simulink model "Day_09_Model_Predictive_Control"  (R2024a)
settings: Solver=FixedStepAuto  StartTime=0.0  StopTime=10  FixedStep=0.01  RelTol=1e-3
values from neighbouring files (symbols this model uses):
  D0 = 2700    [Day_09.m]    (also in Day_09_Method1.m; Day_09_Method2.m)
  D1 = 2700    [Day_09.m]    (also in Day_09_Method1.m; Day_09_Method2.m)
  disturbance = 0.1    [Day_09.m]    (also in Day_09_Method1.m = 0; Day_09_Method2.m = 0)
  L0 = 0.01    [Day_09.m]    (also in Day_09_Method1.m; Day_09_Method2.m)
  L1 = 0.14    [Day_09.m]    (also in Day_09_Method1.m; Day_09_Method2.m)
  limit = inf    [Day_09.m]
  M0 = L0*W0*T0*D0    (= 0.0027)    [Day_09.m]    (also in Day_09_Method1.m; Day_09_Method2.m)
  M1 = L1*W1*T1*D1    (= 0.0378)    [Day_09.m]    (also in Day_09_Method1.m; Day_09_Method2.m)
  M_c = 3    [Day_09.m]    (also in Day_09_Method1.m = 5; Day_09_Method2.m = 5)
  N_p = 10    [Day_09.m]    (also in Day_09_Method1.m = 50; Day_09_Method2.m = 50)
  Q = eye(4)    [Day_09.m]    (also in Day_09_Method1.m = [1 0; 0 1]; Day_09_Method2.m = [1 0; 0 1]; test.m = eye(20))
  R = 1    [Day_09.m]    (also in Day_09_Method1.m; Day_09_Method2.m; test.m = eye(3))
  step_size = 0.01    [Day_09.m]
  T0 = 0.01    [Day_09.m]    (also in Day_09_Method1.m; Day_09_Method2.m)
  T1 = 0.01    [Day_09.m]    (also in Day_09_Method1.m; Day_09_Method2.m)
  W0 = 0.01    [Day_09.m]    (also in Day_09_Method1.m; Day_09_Method2.m)
  W1 = 0.01    [Day_09.m]    (also in Day_09_Method1.m; Day_09_Method2.m)
  x1_d = 0    [Day_09.m]
  x2_d = 0    [Day_09.m]
  x3_d = 0    [Day_09.m]
  x4_d = 0    [Day_09.m]
undefined symbols (not defined in the file or in its folder): X, Y, Z
libraries: sm_lib x14, nesl_utility x7
settings Model: Creator=mingeun  LastModifiedBy=mingeun
settings SolverCC: ZeroCrossAlgorithm=Adaptive
settings DataIOCC: ReturnWorkspaceOutputs=off
settings OptimizationCC: BlockReduction=off  DefaultParameterBehavior=Inlined  BufferReuse=off
settings DebuggingCC: IgnoredZcDiagnostic=none

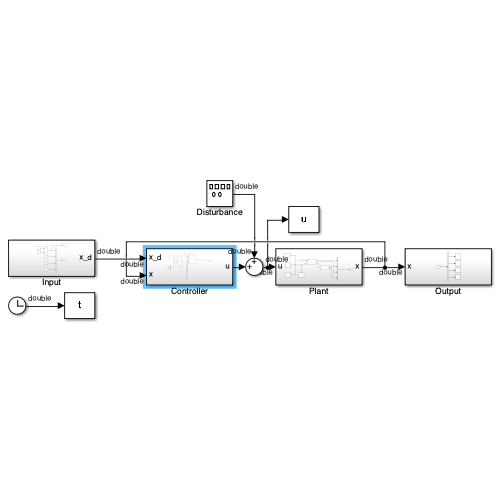
[thumbnail: Simulink's stored preview of the top-level diagram]
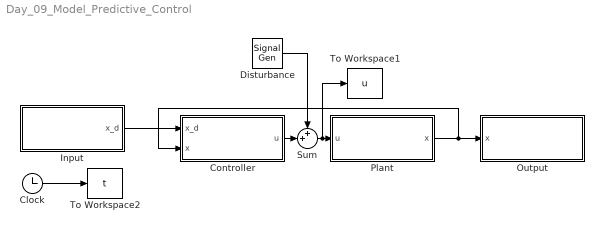
== system Day_09_Model_Predictive_Control ==
  Clock : Clock
  Controller : Subsystem
  Disturbance : SignalGenerator  WaveForm=random  Amplitude=disturbance  Frequency=1e6
  Input : Subsystem
  Output : Subsystem
  Plant : Subsystem
  Sum : Sum  Inputs=++|
  To Workspace1 : ToWorkspace  VariableName=u  SampleTime=-1
  To Workspace2 : ToWorkspace  VariableName=t  SampleTime=-1
  wires:
  Clock/1 -> To Workspace2/1
  Input/1(x_d) -> Controller/1(x_d)
  Plant/1(x) -> Controller/2(x), Output/1(x)
  Controller/1(u) -> Sum/2
  Sum/1 -> To Workspace1/1, Plant/1(u)
  Disturbance/1 -> Sum/1

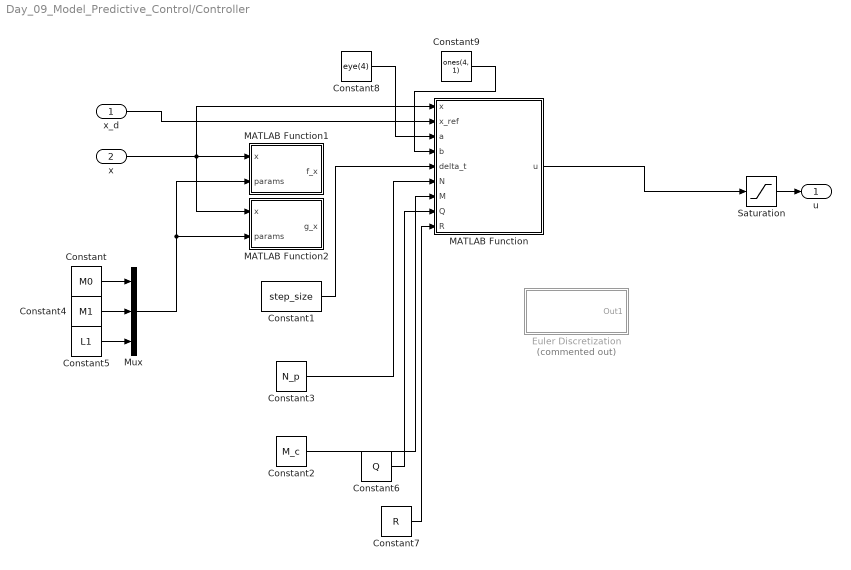
== system Day_09_Model_Predictive_Control/Controller ==
  x_d : Inport
  x : Inport  Port=2
  Constant : Constant  Value=M0
  Constant1 : Constant  Value=step_size
  Constant2 : Constant  Value=M_c
  Constant3 : Constant  Value=N_p
  Constant4 : Constant  Value=M1
  Constant5 : Constant  Value=L1
  Constant6 : Constant  Value=Q
  Constant7 : Constant  Value=R
  Constant8 : Constant  Value=eye(4)
  Constant9 : Constant  Value=ones(4, 1)
  Euler Discretization : Subsystem  Commented=on
  MATLAB Function : MATLAB Function  TreatAsAtomicUnit=on
  MATLAB Function1 : MATLAB Function  TreatAsAtomicUnit=on
  MATLAB Function2 : MATLAB Function  TreatAsAtomicUnit=on
  Mux : Mux  Inputs=3
  Saturation : Saturate  UpperLimit=limit  LowerLimit=-limit
  u : Outport
  wires:
  Saturation/1 -> u/1
  x/1 -> MATLAB Function/1(x), MATLAB Function2/1(x), MATLAB Function1/1(x)
  Constant5/1 -> Mux/3
  Constant4/1 -> Mux/2
  Constant/1 -> Mux/1
  Mux/1 -> MATLAB Function1/2(params), MATLAB Function2/2(params)
  MATLAB Function/1(u) -> Saturation/1
  x_d/1 -> MATLAB Function/2(x_ref)
  Constant1/1 -> MATLAB Function/5(delta_t)
  Constant3/1 -> MATLAB Function/6(N)
  Constant2/1 -> MATLAB Function/7(M)
  Constant6/1 -> MATLAB Function/8(Q)
  Constant7/1 -> MATLAB Function/9(R)
  Constant8/1 -> MATLAB Function/3(a)
  Constant9/1 -> MATLAB Function/4(b)

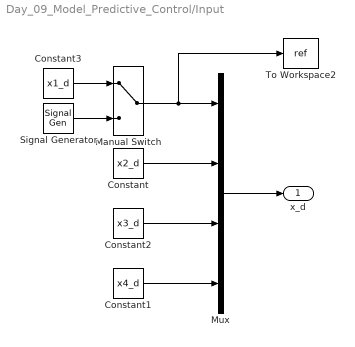
== system Day_09_Model_Predictive_Control/Input ==
  Constant : Constant  Value=x2_d
  Constant1 : Constant  Value=x4_d
  Constant2 : Constant  Value=x3_d
  Constant3 : Constant  Value=x1_d
  Manual Switch : ManualSwitch
  Mux : Mux
  Signal Generator : SignalGenerator  Amplitude=0.2  Units=rad/sec
  To Workspace2 : ToWorkspace  VariableName=ref  SampleTime=-1
  x_d : Outport
  wires:
  Mux/1 -> x_d/1
  Constant/1 -> Mux/2
  Manual Switch/1 -> To Workspace2/1, Mux/1
  Constant2/1 -> Mux/3
  Constant1/1 -> Mux/4
  Signal Generator/1 -> Manual Switch/2
  Constant3/1 -> Manual Switch/1

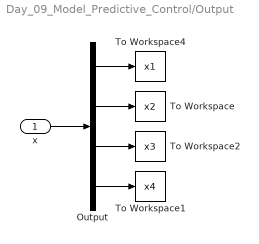
== system Day_09_Model_Predictive_Control/Output ==
  x : Inport
  Output : Demux
  To Workspace : ToWorkspace  VariableName=x2  SampleTime=-1
  To Workspace1 : ToWorkspace  VariableName=x4  SampleTime=-1
  To Workspace2 : ToWorkspace  VariableName=x3  SampleTime=-1
  To Workspace4 : ToWorkspace  VariableName=x1  SampleTime=-1
  wires:
  Output/3 -> To Workspace2/1
  Output/4 -> To Workspace1/1
  Output/2 -> To Workspace/1
  Output/1 -> To Workspace4/1
  x/1 -> Output/1

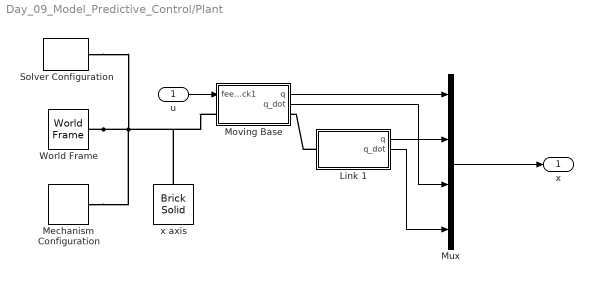
== system Day_09_Model_Predictive_Control/Plant ==
  u : Inport
  Link 1 : Subsystem  mask{L=L1*100, W=W1*100, H=T1*100, rho=D1, rgb=[0.25 0.40 0.70], angle=0, F=0}
      mask prompts: L "Length (cm)"; W "Width (cm)"; H "Thickness (cm)"; rho "Density (kg/m^3)"; rgb "Color [R G B]"; angle "Initial Angle (degree)"; F "Disturbance [N]"
  Mechanism Configuration : sm_lib/Utilities/Mechanism Configuration  UniformGravity=Constant  GravityVector=[0 0 -9.80665]  GravityVectorUnits=m/s^2  LinearizationDelta=0.001  JointModeTransitionNonlinearIterations=2
  Moving Base : Subsystem  mask{L=L0*100, W=W0*100, H=T0*100, rho=D0, RGB=[0.8 0.45 0.0], x_init=0}
      mask prompts: L "Length (cm)"; W "Width (cm)"; H "Thickness (cm)"; rho "Density (kg/m^3)"; RGB "Color [R G B]"; x_init "x_init (cm)"
  Mux : Mux
  Solver Configuration : nesl_utility/Solver Configuration  PhysicalDomain=network_engine_domain  SubClassName=solver  LeftPortType=input  RightPortType=generic  Tones=[]  Harmonics=[]  SimulateNoise=off  Profile=off  UseLocalSampling=off  EnableSwitchedLinearOptims=on  FrequencyDomain=off  UseCCode=off  RelTol=0.001  AbsTol=0.001  MinStep=1e-09  ToWorkspace=off  RevertToSquareIcSolve=off  NumHomotopyIterations=100  PhasorMode=off  PhasorModeNumHarmonics=1  ConsistencySolver=NEWTON_XTOL_AFTER_FTOL  IndexReductionMethod=DerivativeReplacement  DoDC=off  ResidualTolerance=1e-09  ConsistencyTolSource=GLOBAL  ConsistencyAbsTol=0.001  ConsistencyRelTol=0.001  ConsistencyTolFactor=0.001  UseLocalSolver=off  LocalSolverChoice=NE_BACKWARD_EULER_ADVANCER  ResolveIndetEquations=on  FunctionEvalNumThread=1  LocalSolverSampleTime=0.001  DoFixedCost=off  MaxNonlinIter=3  MaxModeIter=2  ComputeImpulses=off  ImpulseIterations=2  LinearAlgebra=auto  LinearAlgebraNumThread=0  EquationFormulation=NE_TIME_EF  DelaysMemoryBudget=1024  AutomaticFiltering=on  FilteringTimeConstant=0.001  PartitionStorageMethod=AS_NEEDED  PartitionMemoryBudget=1024  PartitionMethod=ROBUST  MultibodyUseLocalSolver=off  MultibodyLocalSolverChoice=ODE1  MultibodyLocalSolverSampleTime=0.001
  World Frame : sm_lib/Frames and Transforms/World Frame
  x axis : sm_lib/Body Elements/Brick Solid  BrickDimensions=[1000 1 1]  BrickDimensionsUnits=mm  ExportEntireGeometry=off  InertiaType=CalculateFromGeometry  BasedOnType=Density  Density=1000  DensityUnits=kg/m^3  Mass=1  MassUnits=kg  CenterOfMass=[0 0 0]  CenterOfMassUnits=m  MomentsOfInertia=[1 1 1]  MomentsOfInertiaUnits=kg*m^2  ProductsOfInertia=[0 0 0]  ProductsOfInertiaUnits=kg*m^2  GraphicType=FromGeometry  MarkerShape=Sphere  MarkerSize=10  GraphicVisPropType=SimpleVisualProperties  GraphicDiffuseColor=[0.0 0.0 0.0]  GraphicOpacity=1  GraphicSpecularColor=[0.5 0.5 0.5 1.0]  GraphicAmbientColor=[0.15 0.15 0.15 1.0]  GraphicEmissiveColor=[0.0 0.0 0.0 1.0]  GraphicShininess=75  DoExposeReferenceFrame=on  SerializedFrames=<Frames/>
  x : Outport
  wires:
  Moving Base/1(q) -> Mux/1
  Link 1/1(q) -> Mux/2
  u/1 -> Moving Base/1(feedback1)
  Link 1/2(q_dot) -> Mux/4
  Moving Base/2(q_dot) -> Mux/3
  Mux/1 -> x/1
  connections:
  World Frame/RConn1 -- Solver Configuration/RConn1 -- Moving Base/LConn1 -- x axis/RConn1 -- Mechanism Configuration/RConn1
  Link 1/LConn1 -- Moving Base/RConn1

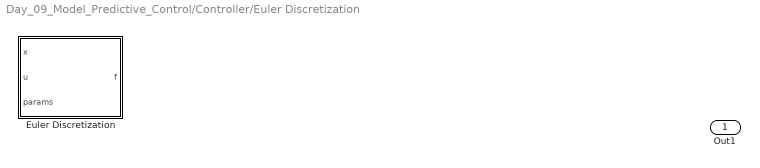
== system Day_09_Model_Predictive_Control/Controller/Euler Discretization ==
  Euler Discretization : MATLAB Function  TreatAsAtomicUnit=on
  Out1 : Outport
  wires:
  ? -> Out1/1

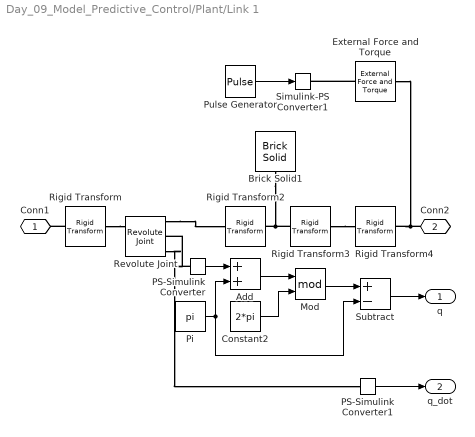
== system Day_09_Model_Predictive_Control/Plant/Link 1 ==
  Add : Sum
  Brick Solid1 : sm_lib/Body Elements/Brick Solid  BrickDimensions=[L W H]  BrickDimensionsUnits=cm  ExportEntireGeometry=off  InertiaType=CalculateFromGeometry  BasedOnType=Density  Density=rho  DensityUnits=kg/m^3  Mass=1  MassUnits=kg  CenterOfMass=[0 0 0]  CenterOfMassUnits=m  MomentsOfInertia=[1 1 1]  MomentsOfInertiaUnits=kg*m^2  ProductsOfInertia=[0 0 0]  ProductsOfInertiaUnits=kg*m^2  GraphicType=FromGeometry  MarkerShape=Sphere  MarkerSize=10  GraphicVisPropType=SimpleVisualProperties  GraphicDiffuseColor=rgb  GraphicOpacity=1  GraphicSpecularColor=[0.5 0.5 0.5 1.0]  GraphicAmbientColor=[0.15 0.15 0.15 1.0]  GraphicEmissiveColor=[0.0 0.0 0.0 1.0]  GraphicShininess=75  DoExposeReferenceFrame=on  SerializedFrames=<Frames/>
  Constant2 : Constant  Value=2*pi
  External Force and Torque : sm_lib/Forces and Torques/External Force and Torque  EnableForceX=on  EnableForceY=off  EnableForceZ=off  EnableForce=off  ForceResolutionFrame=World  EnableTorqueX=off  EnableTorqueY=off  EnableTorqueZ=off  EnableTorque=off  TorqueResolutionFrame=World
  Mod : Math  Operator=mod  OutputSignalType=real
  PS-Simulink Converter : nesl_utility/PS-Simulink Converter  PhysicalDomain=network_engine_domain  SubClassName=ps_output  LeftPortType=input  RightPortType=output  PseudoPeriodic=off  Frequencies=[]  VectorFormat=inherit  Unit=inherit  AffineConversion=off
  PS-Simulink Converter1 : nesl_utility/PS-Simulink Converter  PhysicalDomain=network_engine_domain  SubClassName=ps_output  LeftPortType=input  RightPortType=output  PseudoPeriodic=off  Frequencies=[]  VectorFormat=inherit  Unit=inherit  AffineConversion=off
  Pi : Constant  Value=pi  OutDataTypeStr=Inherit: Inherit via back propagation
  Pulse Generator : DiscretePulseGenerator  PulseType=Time based  Amplitude=F  Period=1000000  PulseWidth=1/1000000  PhaseDelay=0.25
  Revolute Joint : sm_lib/Joints/Revolute Joint  JointMode=Normal  CompositeWrenchDir=FollowerOnBase  CompositeWrenchFrame=BaseFrame  SenseConstraintForce=off  SenseConstraintTorque=off  SenseTotalForce=off  SenseTotalTorque=off  PositionTargetSpecify=on  PositionTargetPriority=High  PositionTargetValue=angle  PositionTargetValueUnits=deg  VelocityTargetSpecify=off  VelocityTargetPriority=High  VelocityTargetValue=0  VelocityTargetValueUnits=deg/s  EquilibriumPosition=0  EquilibriumPositionUnits=deg  SpringStiffness=0  SpringStiffnessUnits=N*m/deg  DampingCoefficient=0  DampingCoefficientUnits=N*m/(deg/s)  LowerLimitSpecify=off  LowerLimitBound=-90  LowerLimitBoundUnits=deg  LowerLimitStiffness=1e4  LowerLimitStiffnessUnits=N*m/deg  LowerLimitDamping=10  LowerLimitDampingUnits=N*m/(deg/s)  LowerLimitTransitionRegionWidth=0.1  LowerLimitTransitionRegionWidthUnits=deg  UpperLimitSpecify=off  UpperLimitBound=90  UpperLimitBoundUnits=deg  UpperLimitStiffness=1e4  UpperLimitStiffnessUnits=N*m/deg  UpperLimitDamping=10  UpperLimitDampingUnits=N*m/(deg/s)  UpperLimitTransitionRegionWidth=0.1  UpperLimitTransitionRegionWidthUnits=deg  TorqueActuationMode=InputTorque  MotionActuationMode=ComputedMotion  SensePosition=on  SenseVelocity=on  SenseAcceleration=off  SenseTorqueForce=off  SenseLowerLimitTorqueForce=off  SenseUpperLimitTorqueForce=off
  Rigid Transform : sm_lib/Frames and Transforms/Rigid Transform  RotationMethod=RotationMatrix  FollAlignAxisA=+X  BaseAlignAxisA=+Y  FollAlignAxisB=+Y  BaseAlignAxisB=+Z  RotationStandardAxis=+X  RotationAngle=90  RotationAngleUnits=deg  RotationArbitraryAxis=[0 0 1]  RotationSequenceAxes=FollowerAxes  RotationSequence=XYX  RotationSequenceAngles=[0 0 0]  RotationSequenceAnglesUnits=deg  RotationMatrix=[0 0 1; -1 0 0; 0 -1 0]  Quaternion=[1 0 0 0]  TranslationMethod=None  TranslationCartesianOffset=[0 0 0]  TranslationCartesianOffsetUnits=m  TranslationStandardAxis=+Z  TranslationStandardOffset=0  TranslationStandardOffsetUnits=m  TranslationROffset=0  TranslationROffsetUnits=m  TranslationThetaOffset=0  TranslationThetaOffsetUnits=deg  TranslationZOffset=0  TranslationZOffsetUnits=m
  Rigid Transform2 : sm_lib/Frames and Transforms/Rigid Transform  RotationMethod=None  FollAlignAxisA=+X  BaseAlignAxisA=+Y  FollAlignAxisB=+Y  BaseAlignAxisB=+Z  RotationStandardAxis=+Z  RotationAngle=0  RotationAngleUnits=deg  RotationArbitraryAxis=[0 0 1]  RotationSequenceAxes=FollowerAxes  RotationSequence=XYX  RotationSequenceAngles=[0 0 0]  RotationSequenceAnglesUnits=deg  RotationMatrix=[1 0 0;0 1 0;0 0 1]  Quaternion=[1 0 0 0]  TranslationMethod=StandardAxis  TranslationCartesianOffset=[0 0 0]  TranslationCartesianOffsetUnits=m  TranslationStandardAxis=-X  TranslationStandardOffset=L/2  TranslationStandardOffsetUnits=cm  TranslationROffset=0  TranslationROffsetUnits=m  TranslationThetaOffset=0  TranslationThetaOffsetUnits=deg  TranslationZOffset=0  TranslationZOffsetUnits=m
  Rigid Transform3 : sm_lib/Frames and Transforms/Rigid Transform  RotationMethod=None  FollAlignAxisA=+X  BaseAlignAxisA=+Y  FollAlignAxisB=+Y  BaseAlignAxisB=+Z  RotationStandardAxis=+Z  RotationAngle=0  RotationAngleUnits=deg  RotationArbitraryAxis=[0 0 1]  RotationSequenceAxes=FollowerAxes  RotationSequence=XYX  RotationSequenceAngles=[0 0 0]  RotationSequenceAnglesUnits=deg  RotationMatrix=[1 0 0;0 1 0;0 0 1]  Quaternion=[1 0 0 0]  TranslationMethod=StandardAxis  TranslationCartesianOffset=[0 0 0]  TranslationCartesianOffsetUnits=m  TranslationStandardAxis=-X  TranslationStandardOffset=L/2  TranslationStandardOffsetUnits=cm  TranslationROffset=0  TranslationROffsetUnits=m  TranslationThetaOffset=0  TranslationThetaOffsetUnits=deg  TranslationZOffset=0  TranslationZOffsetUnits=m
  Rigid Transform4 : sm_lib/Frames and Transforms/Rigid Transform  RotationMethod=None  FollAlignAxisA=+X  BaseAlignAxisA=+Y  FollAlignAxisB=+Y  BaseAlignAxisB=+Z  RotationStandardAxis=+Z  RotationAngle=0  RotationAngleUnits=deg  RotationArbitraryAxis=[0 0 1]  RotationSequenceAxes=FollowerAxes  RotationSequence=XYX  RotationSequenceAngles=[0 0 0]  RotationSequenceAnglesUnits=deg  RotationMatrix=[1 0 0; 0 0 1; 0 -1 0]  Quaternion=[1 0 0 0]  TranslationMethod=StandardAxis  TranslationCartesianOffset=[0 0 0]  TranslationCartesianOffsetUnits=m  TranslationStandardAxis=+X  TranslationStandardOffset=L  TranslationStandardOffsetUnits=cm  TranslationROffset=0  TranslationROffsetUnits=m  TranslationThetaOffset=0  TranslationThetaOffsetUnits=deg  TranslationZOffset=0  TranslationZOffsetUnits=m
  Simulink-PS Converter1 : nesl_utility/Simulink-PS Converter  PhysicalDomain=network_engine_domain  SubClassName=ps_input  LeftPortType=input  RightPortType=output  PseudoPeriodic=off  Frequencies=[]  NoiseDistribution=none  NoiseParameters=[]  Unit=1  AffineConversion=off  FilteringAndDerivatives=provide  SimscapeFilterOrder=1  InputFilterTimeConstant=0.001  UdotUserProvided=0
  Subtract : Sum  Inputs=+-
  Conn1 : PMIOPort  Side=Left
  Conn2 : PMIOPort  Port=2  Side=Right
  q : Outport
  q_dot : Outport  Port=2
  wires:
  Pulse Generator/1 -> Simulink-PS Converter1/1
  Mod/1 -> Subtract/1
  Constant2/1 -> Mod/2
  Pi/1 -> Subtract/2, Add/2
  PS-Simulink Converter/1 -> Add/1
  Add/1 -> Mod/1
  Subtract/1 -> q/1
  PS-Simulink Converter1/1 -> q_dot/1
  connections:
  PS-Simulink Converter/LConn1 -- Revolute Joint/RConn2
  Rigid Transform3/RConn1 -- Rigid Transform4/LConn1
  Rigid Transform/LConn1 -- Revolute Joint/LConn1
  Rigid Transform3/LConn1 -- Brick Solid1/RConn1 -- Rigid Transform2/LConn1
  Conn2/RConn1 -- External Force and Torque/RConn1 -- Rigid Transform4/RConn1
  Rigid Transform/RConn1 -- Conn1/RConn1
  Revolute Joint/RConn1 -- Rigid Transform2/RConn1
  External Force and Torque/LConn1 -- Simulink-PS Converter1/RConn1
  Revolute Joint/RConn3 -- PS-Simulink Converter1/LConn1

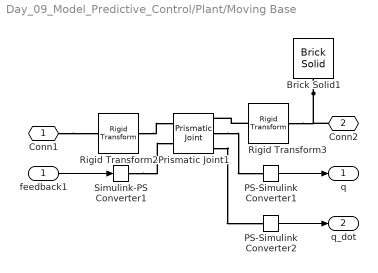
== system Day_09_Model_Predictive_Control/Plant/Moving Base ==
  feedback1 : Inport
  Brick Solid1 : sm_lib/Body Elements/Brick Solid  BrickDimensions=[L W H]  BrickDimensionsUnits=cm  ExportEntireGeometry=off  InertiaType=CalculateFromGeometry  BasedOnType=Density  Density=rho  DensityUnits=kg/m^3  Mass=1  MassUnits=kg  CenterOfMass=[0 0 0]  CenterOfMassUnits=m  MomentsOfInertia=[1 1 1]  MomentsOfInertiaUnits=kg*m^2  ProductsOfInertia=[0 0 0]  ProductsOfInertiaUnits=kg*m^2  GraphicType=FromGeometry  MarkerShape=Sphere  MarkerSize=10  GraphicVisPropType=SimpleVisualProperties  GraphicDiffuseColor=RGB  GraphicOpacity=1  GraphicSpecularColor=[0.5 0.5 0.5 1.0]  GraphicAmbientColor=[0.15 0.15 0.15 1.0]  GraphicEmissiveColor=[0.0 0.0 0.0 1.0]  GraphicShininess=75  DoExposeReferenceFrame=on  SerializedFrames=<Frames/>
  PS-Simulink Converter1 : nesl_utility/PS-Simulink Converter  PhysicalDomain=network_engine_domain  SubClassName=ps_output  LeftPortType=input  RightPortType=output  PseudoPeriodic=off  Frequencies=[]  VectorFormat=inherit  Unit=inherit  AffineConversion=off
  PS-Simulink Converter2 : nesl_utility/PS-Simulink Converter  PhysicalDomain=network_engine_domain  SubClassName=ps_output  LeftPortType=input  RightPortType=output  PseudoPeriodic=off  Frequencies=[]  VectorFormat=inherit  Unit=inherit  AffineConversion=off
  Prismatic Joint1 : sm_lib/Joints/Prismatic Joint  JointMode=Normal  CompositeWrenchDir=FollowerOnBase  CompositeWrenchFrame=BaseFrame  SenseConstraintForce=off  SenseConstraintTorque=off  SenseTotalForce=off  SenseTotalTorque=off  PositionTargetSpecify=on  PositionTargetPriority=High  PositionTargetValue=x_init  PositionTargetValueUnits=cm  VelocityTargetSpecify=off  VelocityTargetPriority=High  VelocityTargetValue=0  VelocityTargetValueUnits=m/s  EquilibriumPosition=0  EquilibriumPositionUnits=m  SpringStiffness=0  SpringStiffnessUnits=N/m  DampingCoefficient=0  DampingCoefficientUnits=N/(m/s)  LowerLimitSpecify=off  LowerLimitBound=-1  LowerLimitBoundUnits=m  LowerLimitStiffness=1e6  LowerLimitStiffnessUnits=N/m  LowerLimitDamping=1e3  LowerLimitDampingUnits=N/(m/s)  LowerLimitTransitionRegionWidth=1e-4  LowerLimitTransitionRegionWidthUnits=m  UpperLimitSpecify=off  UpperLimitBound=1  UpperLimitBoundUnits=m  UpperLimitStiffness=1e6  UpperLimitStiffnessUnits=N/m  UpperLimitDamping=1e3  UpperLimitDampingUnits=N/(m/s)  UpperLimitTransitionRegionWidth=1e-4  UpperLimitTransitionRegionWidthUnits=m  TorqueActuationMode=InputTorque  MotionActuationMode=ComputedMotion  SensePosition=on  SenseVelocity=on  SenseAcceleration=off  SenseTorqueForce=off  SenseLowerLimitTorqueForce=off  SenseUpperLimitTorqueForce=off
  Rigid Transform2 : sm_lib/Frames and Transforms/Rigid Transform  RotationMethod=StandardAxis  FollAlignAxisA=+X  BaseAlignAxisA=+Y  FollAlignAxisB=+Y  BaseAlignAxisB=+Z  RotationStandardAxis=+Y  RotationAngle=90  RotationAngleUnits=deg  RotationArbitraryAxis=[0 0 1]  RotationSequenceAxes=FollowerAxes  RotationSequence=XYX  RotationSequenceAngles=[0 0 0]  RotationSequenceAnglesUnits=deg  RotationMatrix=[1 0 0;0 1 0;0 0 1]  Quaternion=[1 0 0 0]  TranslationMethod=None  TranslationCartesianOffset=[0 0 0]  TranslationCartesianOffsetUnits=m  TranslationStandardAxis=+Z  TranslationStandardOffset=0  TranslationStandardOffsetUnits=m  TranslationROffset=0  TranslationROffsetUnits=m  TranslationThetaOffset=0  TranslationThetaOffsetUnits=deg  TranslationZOffset=0  TranslationZOffsetUnits=m
  Rigid Transform3 : sm_lib/Frames and Transforms/Rigid Transform  RotationMethod=StandardAxis  FollAlignAxisA=+X  BaseAlignAxisA=+Y  FollAlignAxisB=+Y  BaseAlignAxisB=+Z  RotationStandardAxis=+Y  RotationAngle=90  RotationAngleUnits=deg  RotationArbitraryAxis=[0 0 1]  RotationSequenceAxes=FollowerAxes  RotationSequence=XYX  RotationSequenceAngles=[0 0 0]  RotationSequenceAnglesUnits=deg  RotationMatrix=[1 0 0;0 1 0;0 0 1]  Quaternion=[1 0 0 0]  TranslationMethod=None  TranslationCartesianOffset=[0 0 0]  TranslationCartesianOffsetUnits=m  TranslationStandardAxis=+Z  TranslationStandardOffset=0  TranslationStandardOffsetUnits=m  TranslationROffset=0  TranslationROffsetUnits=m  TranslationThetaOffset=0  TranslationThetaOffsetUnits=deg  TranslationZOffset=0  TranslationZOffsetUnits=m
  Simulink-PS Converter1 : nesl_utility/Simulink-PS Converter  PhysicalDomain=network_engine_domain  SubClassName=ps_input  LeftPortType=input  RightPortType=output  PseudoPeriodic=off  Frequencies=[]  NoiseDistribution=none  NoiseParameters=[]  Unit=1  AffineConversion=off  FilteringAndDerivatives=provide  SimscapeFilterOrder=1  InputFilterTimeConstant=0.001  UdotUserProvided=0
  Conn1 : PMIOPort  Side=Left
  Conn2 : PMIOPort  Port=2  Side=Right
  q : Outport
  q_dot : Outport  Port=2
  wires:
  feedback1/1 -> Simulink-PS Converter1/1
  PS-Simulink Converter1/1 -> q/1
  PS-Simulink Converter2/1 -> q_dot/1
  connections:
  Brick Solid1/RConn1 -- Conn2/RConn1 -- Rigid Transform3/LConn1
  Rigid Transform2/RConn1 -- Prismatic Joint1/LConn1
  Prismatic Joint1/RConn2 -- PS-Simulink Converter1/LConn1
  Simulink-PS Converter1/RConn1 -- Prismatic Joint1/LConn2
  Conn1/RConn1 -- Rigid Transform2/LConn1
  Rigid Transform3/RConn1 -- Prismatic Joint1/RConn1
  Prismatic Joint1/RConn3 -- PS-Simulink Converter2/LConn1

== matlab function Day_09_Model_Predictive_Control/Controller/MATLAB Function1 ==
  data: x input; f_x output; params input
function f_x = fcn(x, params)
x1 = x(1);
x2 = x(2);
x3 = x(3);
x4 = x(4);

m0 = params(1);
m1 = params(2);
l1 = params(3);

g = 9.81;

f_x = [x3;
       x4;
       (m1*sin(x2)*(3*g*cos(x2) - 2*l1*x4^2))/(4*m0 + 4*m1 - 3*m1*cos(x2)^2);
       (3*sin(x2)*(2*g*m0 + 2*g*m1 - l1*m1*cos(x2)*x4^2))/(l1*(4*m0 + 4*m1 - 3*m1*cos(x2)^2))];

== matlab function Day_09_Model_Predictive_Control/Controller/Euler Discretization/Euler Discretization ==
  data: x input; u input; f output; params input
function f = fcn(x, u, params)
x2 = x(2);
x3 = x(3);
x4 = x(4);

m0 = params(1);
m1 = params(2);
l1 = params(3);

g = 9.81;

PH = zeros(4, N + 1);
PH(:, 1) = x;

for i = 1 : N
f = [x3;
     x4;
     (4*u - 2*l1*m1*sin(x2)*x4^2 + 3*g*m1*cos(x2)*sin(x2))/(4*m0 + 4*m1 - 3*m1*cos(x2)^2);
     (6*cos(x2)*(u - (l1*m1*sin(x2)*x4^2)/2))/(4*l1*m0 + 4*l1*m1 - 3*l1*m1*cos(x2)^2) + (6*g*l1*m1*sin(x2)*(m0 + m1))/(4*l1^2*m1^2 + 4*l1^2*m0*m1 - 3*l1^2*m1^2*cos(x2)^2)];

PH(:, i + 1) = PH(:, i) + dt * f;
x2 = PH(2, i+1);
x3 = PH(3, i+1);
x4 = PH(4, i+1);
end

PH = PH(2:end, :);

== matlab function Day_09_Model_Predictive_Control/Controller/MATLAB Function2 ==
  data: x input; g_x output; params input
function g_x = fcn(x, params)
x1 = x(1);
x2 = x(2);
x3 = x(3);
x4 = x(4);

m0 = params(1);
m1 = params(2);
l1 = params(3);

g = 9.81;

g_x = [0;
       0;
       4/(4*m0 + 4*m1 - 3*m1*cos(x2)^2);
       (6*cos(x2))/(4*l1*m0 + 4*l1*m1 - 3*l1*m1*cos(x2)^2)];

== matlab function Day_09_Model_Predictive_Control/Controller/MATLAB Function ==
  data: x input; x_ref input; u output; a input; b input; delta_t input; N input; M input; Q input; R input
function u = mpc_sqp(x, x_ref, a, b, delta_t, N, M, Q, R)
% MPC controller using SQP method

% Initial guess for control input sequence (only first M are optimized)
u_initial = zeros(M, 1);

% Setup optimization parameters
max_iters = 10; % Maximum iterations for SQP
tolerance = 1e-6;

% Initialize SQP loop
u_opt = u_initial;
lambda = zeros(M, 1); % Initialize Lagrange multipliers
for iter = 1:max_iters
    % 1. Linearize the cost function and constraints
    [H, g] = compute_quadratic_approximation(x, x_ref, u_opt, a, b, delta_t, N, M, Q, R);
    
    % 2. Solve the quadratic programming (QP) subproblem
    options = optimoptions('quadprog', 'Algorithm', 'active-set', 'Display', 'off');
    u_new = quadprog(H, g, [], [], [], [], -1*ones(M,1), 1*ones(M,1), u_initial, options);
    
    % 3. Update solution and check for convergence
    if norm(u_new - u_opt) < tolerance
        break;
    end
    u_opt = u_new;
end

% Return the first control input
u = u_opt(1);
end

function [H, g] = compute_quadratic_approximation(x, x_ref, u_opt, a, b, delta_t, N, M, Q, R)
% Compute the Hessian (H) and gradient (g) for the QP subproblem

H = zeros(M, M);
g = zeros(M, 1);
x_k = x;

for i = 1:N
    if i <= M
        u_k = u_opt(i);
    else
        u_k = u_opt(M); % Use the last control input for i > M
    end
    
    % Predict next state
    x_k = x_k + delta_t * (a * x_k + b * u_k);
    
    % Compute gradient g and Hessian H for QP
    g(i) = 2 * (delta_t * a * (x_k - x_ref))' * Q * (delta_t * a * (x_k - x_ref)) + 2 * R * u_k;
    if i <= M
        H(i, i) = 2 * delta_t^2 * trace(a' * Q * a) + 2 * R;
    end
end
end
